simulink model "ChildsPhone_fuzzyLogic"  (R2024a)
settings: Solver=FixedStepAuto  StartTime=0.0  StopTime=inf  RelTol=1e-3
undefined symbols (not defined in the file): Altitude, ChildPhone, Danger_Level, Latitude, Longitude, mic, My_Sound, Voice, Z
libraries: androidcommunicationlib x4, androiduilib x4, androidaudiovideolib x3, androidsensorlib x2, fuzblock x1
settings Model: Creator=Omkar R Prabhu  LastModifiedBy=Omkar R Prabhu
settings OptimizationCC: EnhancedBackFolding=on  PassReuseOutputArgsAs=Individual arguments  ZeroExternalMemoryAtStartup=off  ZeroInternalMemoryAtStartup=off  MaxStackSize=64  OptimizeBlockOrder=speed  DifferentSizesBufferReuse=on  OptimizationCustomize=off  EfficientTunableParamExpr=on
settings DebuggingCC: ParameterTunabilityLossMsg=error
settings HardwareCC: ProdBitPerPointer=32  ProdBitPerSizeT=32  ProdBitPerPtrDiffT=32  ProdLargestAtomicInteger=Long  ProdLargestAtomicFloat=Double  ProdWordSize=32  ProdHWDeviceType=ARM Compatible->ARM Cortex  UseEmbeddedCoderFeatures=off  UseSimulinkCoderFeatures=off
settings SFSimCC: MATLABDynamicMemAlloc=off
settings RTWCC: Description=Embedded Coder  SystemTargetFile=ert.tlc  HardwareBoard=Android Device  TLCOptions="-aInlineSetEventsForThisBaseRateFcn=TLC_FALSE -aSuppressMultiTaskScheduler=TLC_FALSE  -aRateBasedStepFcn=0"  TemplateMakefile=ert_default_tmf  RTWVerbose=off  Toolchain=Android SDK/NDK Tools
settings CodeAppCC: ForceParamTrailComments=on  IgnoreCustomStorageClasses=off  OperatorAnnotations=on  SimulinkDataObjDesc=on  SFDataObjDesc=on  InsertBlockDesc=on
settings ERTTargetCC: SupportNonInlinedSFcns=on

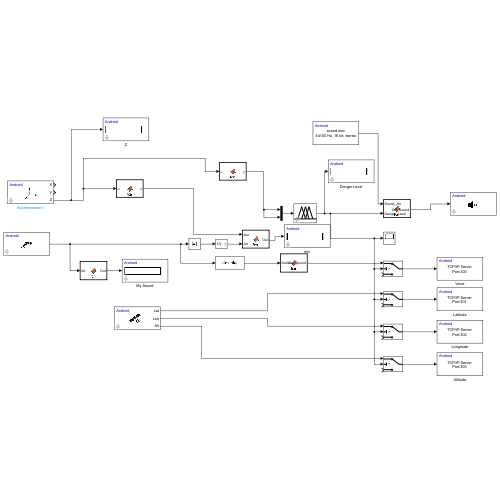
[thumbnail: Simulink's stored preview of the top-level diagram]
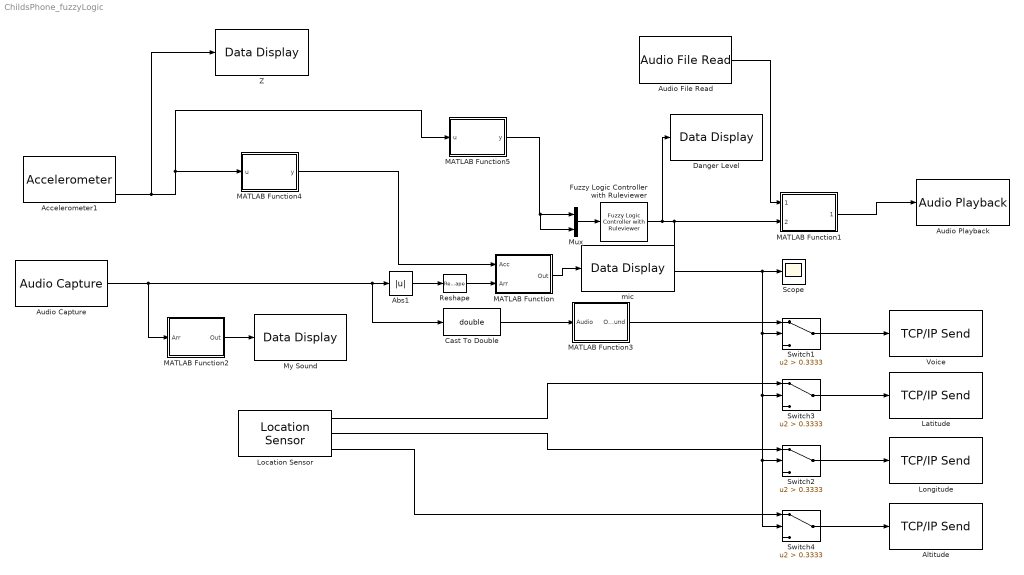
== system ChildsPhone_fuzzyLogic ==
  Abs1 : Abs  SaturateOnIntegerOverflow=off
  Accelerometer1 : androidsensorlib/Accelerometer  OutputVector=off  SampleTime=0.1  BlockPlatform=Android
  Altitude : androidcommunicationlib/TCP//IP Send  TCPSendId=ChildPhone/Altitude  Mode_=Server  LocalServerPort_=303  RemoteAddr_=127.0.0.4  RemoteServerPort_=25000  ClientPortBindingSelection_=off  ClientPortToBind_=35000  BlockingMode_=off  BlockTimeout_=0.1
  Audio Capture : androidaudiovideolib/Audio Capture  SampleFreq=44100  FrameSize=4410  SampleTime=0.1  SimulateUsing=Code generation  DeviceStr=0  QueueDuration=0  BlockPlatform=Android  AudioSamplingFreq=44100
  Audio File Read : androidaudiovideolib/Audio File Read  FileName=C:\kd\sound.wav  FrameSize=4410
  Audio Playback : androidaudiovideolib/Audio Playback  SampleFreq=44100  AudioSamplingFreq=44100  SampleTime=0.1  DeviceStr=0  QueueDuration=0  BlockPlatform=Android
  Cast To Double : DataTypeConversion  OutDataTypeStr=double  SaturateOnIntegerOverflow=off  RndMeth=Floor
  Danger Level : androiduilib/Data Display  DataDisplayId=ChildPhone/Danger_Level  Format=Float  Precision=6  SimulateUsing=Code generation  blockPlatform=Android
  Fuzzy Logic Controller with Ruleviewer : fuzblock/Fuzzy Logic  Controller  with Ruleviewer  fismatrix=mamdanitype1  Ts=2
  Latitude : androidcommunicationlib/TCP//IP Send  TCPSendId=ChildPhone/Latitude  Mode_=Server  LocalServerPort_=301  RemoteAddr_=127.0.0.2  RemoteServerPort_=25000  ClientPortBindingSelection_=off  ClientPortToBind_=35000  BlockingMode_=off  BlockTimeout_=0.1
  Location Sensor : androidsensorlib/Location Sensor  OutputVector=off  SampleTime=0.1  BlockPlatform=Android
  Longitude : androidcommunicationlib/TCP//IP Send  TCPSendId=ChildPhone/Longitude  Mode_=Server  LocalServerPort_=302  RemoteAddr_=127.0.0.3  RemoteServerPort_=25000  ClientPortBindingSelection_=off  ClientPortToBind_=35000  BlockingMode_=off  BlockTimeout_=0.1
  MATLAB Function : MATLAB Function  TreatAsAtomicUnit=on
  MATLAB Function1 : MATLAB Function  TreatAsAtomicUnit=on
  MATLAB Function2 : MATLAB Function  TreatAsAtomicUnit=on
  MATLAB Function3 : MATLAB Function  TreatAsAtomicUnit=on
  MATLAB Function4 : MATLAB Function  TreatAsAtomicUnit=on
  MATLAB Function5 : MATLAB Function  TreatAsAtomicUnit=on
  Mux : Mux  Inputs=2
  My Sound : androiduilib/Data Display  DataDisplayId=ChildPhone/My_Sound  Format=Float  Precision=6  SimulateUsing=Code generation  blockPlatform=Android
  Reshape : Reshape
  Scope : Scope
  Switch1 : Switch  Criteria=u2 > Threshold  Threshold=0.3333  OutDataTypeStr=double  SaturateOnIntegerOverflow=off  InputSameDT=off
  Switch2 : Switch  Criteria=u2 > Threshold  Threshold=0.3333  SaturateOnIntegerOverflow=off  InputSameDT=off
  Switch3 : Switch  Criteria=u2 > Threshold  Threshold=0.3333  SaturateOnIntegerOverflow=off  InputSameDT=off
  Switch4 : Switch  Criteria=u2 > Threshold  Threshold=0.3333  SaturateOnIntegerOverflow=off  InputSameDT=off
  Voice : androidcommunicationlib/TCP//IP Send  TCPSendId=ChildPhone/Voice  Mode_=Server  LocalServerPort_=300  RemoteAddr_=127.0.0.2  RemoteServerPort_=25000  ClientPortBindingSelection_=off  ClientPortToBind_=35000  BlockingMode_=off  BlockTimeout_=0.1
  Z : androiduilib/Data Display  DataDisplayId=ChildPhone/Z  Format=Float  Precision=6  SimulateUsing=Code generation  blockPlatform=Android
  mic : androiduilib/Data Display  DataDisplayId=ChildPhone/mic  Format=Float  Precision=6  SimulateUsing=Code generation  blockPlatform=Android
  wires:
  MATLAB Function1/1(Out_Sound) -> Audio Playback/1
  Switch3/1 -> Latitude/1
  Switch2/1 -> Longitude/1
  Location Sensor/1 -> Switch3/1
  Audio File Read/1 -> MATLAB Function1/1(Sound_Arr)
  Mux/1 -> Fuzzy Logic Controller with Ruleviewer/1
  Abs1/1 -> Reshape/1
  Reshape/1 -> MATLAB Function/2(Arr)
  MATLAB Function/1(Out) -> mic/1
  Audio Capture/1 -> MATLAB Function2/1(Arr), Cast To Double/1, Abs1/1
  Location Sensor/2 -> Switch2/1
  Switch4/1 -> Altitude/1
  Location Sensor/3 -> Switch4/1
  Fuzzy Logic Controller with Ruleviewer/1 -> Danger Level/1, Scope/1, Switch1/2, Switch3/2, Switch4/2, Switch2/2, MATLAB Function1/2(Danger_Level)
  MATLAB Function2/1(Out) -> My Sound/1
  Switch1/1 -> Voice/1
  Cast To Double/1 -> MATLAB Function3/1(Audio)
  MATLAB Function3/1(Out_Sound) -> Switch1/1
  MATLAB Function4/1(y) -> MATLAB Function/1(Acc)
  Accelerometer1/3 -> Z/1, MATLAB Function5/1(u), MATLAB Function4/1(u)
  MATLAB Function5/1(y) -> Mux/2, Mux/1

== matlab function ChildsPhone_fuzzyLogic/MATLAB Function1 ==
  data: Sound_Arr input; Danger_Level input; Out_Sound output
function Out_Sound = fcn(Sound_Arr , Danger_Level)
    if(Danger_Level <= 0.333333)
        Out_Sound = Sound_Arr.*0 ; 
    else if (Danger_Level <= 0.6666)
        Out_Sound = Sound_Arr.*0.1 ;
    else 
        Out_Sound = Sound_Arr ; 
        end
    end 
end

== matlab function ChildsPhone_fuzzyLogic/MATLAB Function2 ==
  data: Arr input; Out output
function Out = fcn(Arr)
    Out = single(max(Arr)) ; 
end

== matlab function ChildsPhone_fuzzyLogic/MATLAB Function3 ==
  data: Audio input; Out_Sound output
function Out_Sound = fcn(Audio)
    Out_Sound  = Audio(:,1) ;
end

== matlab function ChildsPhone_fuzzyLogic/MATLAB Function4 ==
  data: u input; y output
function y = fcn(u)

% Specify y as single data type
y = single(u);

if u < 4
    y = single(1); % Use single() to specify the data type
else
    y = single(0); % Use single() to specify the data type
end

== matlab function ChildsPhone_fuzzyLogic/MATLAB Function5 ==
  data: u input; y output
function y = fcn(u)

y = 10-u;

== matlab function ChildsPhone_fuzzyLogic/MATLAB Function ==
  data: Acc input; Arr input; Out output
function Out = fcn(Acc , Arr)
    if(Acc == 1)
        Out = single(max(Arr)) ; 
    else 
        Out = single(0) ; 
    end 
end
